simulink model "abdoulkader_simulation"  (R2017b)
settings: Solver=VariableStepAuto  StartTime=0.0  StopTime=10.0  RelTol=1e-3
settings Model: Creator=abdoul kader  LastModifiedBy=abdoul kader

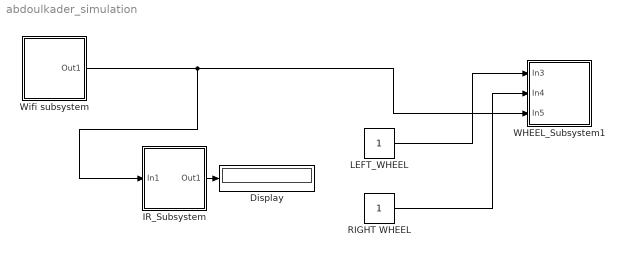
== system abdoulkader_simulation ==
  Display : Display
  IR_Subsystem : Subsystem
  LEFT_WHEEL : Constant
  RIGHT WHEEL : Constant
  WHEEL_Subsystem1 : Subsystem
  Wifi subsystem : Subsystem
  wires:
  LEFT_WHEEL/1 -> WHEEL_Subsystem1/1(In3)
  RIGHT WHEEL/1 -> WHEEL_Subsystem1/2(In4)
  Wifi subsystem/1(Out1) -> WHEEL_Subsystem1/3(In5), IR_Subsystem/1(In1)
  IR_Subsystem/1(Out1) -> Display/1

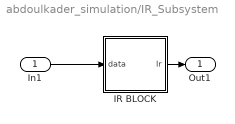
== system abdoulkader_simulation/IR_Subsystem ==
  In1 : Inport
  IR BLOCK : Stateflow chart  TreatAsAtomicUnit=on
  Out1 : Outport
  wires:
  IR BLOCK/1(Ir) -> Out1/1
  In1/1 -> IR BLOCK/1(data)

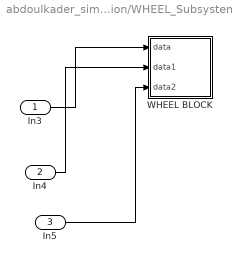
== system abdoulkader_simulation/WHEEL_Subsystem1 ==
  In3 : Inport
  In4 : Inport  Port=2
  In5 : Inport  Port=3
  WHEEL BLOCK : Stateflow chart  TreatAsAtomicUnit=on
  wires:
  In3/1 -> WHEEL BLOCK/1(data)
  In4/1 -> WHEEL BLOCK/2(data1)
  In5/1 -> WHEEL BLOCK/3(data2)

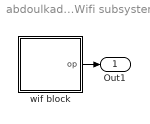
== system abdoulkader_simulation/Wifi subsystem ==
  wif block : Stateflow chart  TreatAsAtomicUnit=on
  Out1 : Outport
  wires:
  wif block/1(op) -> Out1/1

== stateflow chart abdoulkader_simulation/IR_Subsystem/IR BLOCK ==
  state tf
    en,du:
    Ir=IRA;
  data: Ir output; data input
  function IR:
    | function IR
    | y=[0,0,0,0,0,0,];
    | persistent obj
    | coder.extrinsic('evalin');
    | coder.extrinsic('get');
    | if isempty(obj)
    |     obj=evalin('base','re');
    | end
    | coder.extrinsic('RangeStateRoomba');
    | y=RangeStateRoomba(obj);

== stateflow chart abdoulkader_simulation/WHEEL_Subsystem1/WHEEL BLOCK ==
  state kader
    entry,during:
    motor(right,left)
  data: u1 function_input; u2 function_input; data input; data1 input; data2 input
  function motor(u1,u2):
    | function motor(u1,u2)
    | persistent obj
    | coder.extrinsic('RoomBaWiFi')
    | coder.extrinsic('assignin');
    | if isempty(obj)
    |     obj=RoomBaWiFi('10.0.0.1','full')
    | end
    | assignin('base','re',obj)

== stateflow chart abdoulkader_simulation/Wifi subsystem/wif block ==
  state b
    entry,during:
    wifi;
    op=0;
  data: op output
  function wifi:
    | function wifi
    | persistent obj
    | coder.extrinsic('RoomBaWiFi')
    | coder.extrinsic('assignin');
    | if isempty(obj)
    |     obj=RoomBaWiFi('10.0.0.1','full')
    | end
    | assignin('base','re',obj)
